simulink model "BerylMambo"  (R2019b)
settings: Solver=FixedStepAuto  StartTime=0.0  StopTime=100  FixedStep=1/200  RelTol=1e-3
InitFcn:
  | load('BusDefinitions.mat')
undefined symbols (not defined in the file or in its folder): codertarget, DiscIntNeverNeededParam, Discrete, sigbuilder_block, Time
libraries: dspstat3 x7, simulink x5, parrotlib x2, ctrlSharedLib x1
settings Model: SimulationMode=external  ExtModeTrigDuration=80  Creator=kelvinxie  LastModifiedBy=kelvinxie
settings OptimizationCC: PassReuseOutputArgsThreshold=0  MaxStackSize=64  SimCompilerOptimization=on
settings DebuggingCC: ParameterTunabilityLossMsg=error  ArithmeticOperatorsInVariantConditions=warning
settings HardwareCC: ProdBitPerPointer=32  ProdBitPerSizeT=32  ProdBitPerPtrDiffT=32  ProdLargestAtomicInteger=Long  ProdWordSize=32  ProdHWDeviceType=ARM Compatible->ARM 9
settings SFSimCC: SimUseLocalCustomCode=off  MATLABDynamicMemAlloc=off
settings RTWCC: SystemTargetFile=ert.tlc  HardwareBoard=PARROT Mambo  TLCOptions="-aInlineSetEventsForThisBaseRateFcn=TLC_FALSE -aSuppressMultiTaskScheduler=TLC_FALSE   -aRateBasedStepFcn=1"  TemplateMakefile=ert_default_tmf  GenerateReport=on  RTWVerbose=off  RTWUseLocalCustomCode=off  Toolchain=Sourcery G++ Lite GNU Toolchain for Drones  BuildConfiguration=Faster Runs
settings CodeAppCC: ForceParamTrailComments=on  OperatorAnnotations=on  StateflowObjectComments=on
settings ERTTargetCC: ERTCustomFileBanners=off  MatFileLogging=on  SupportContinuousTime=on  SupportNonInlinedSFcns=on  RemoveResetFunc=off  ModelStepFunctionPrototypeControlCompliant=off

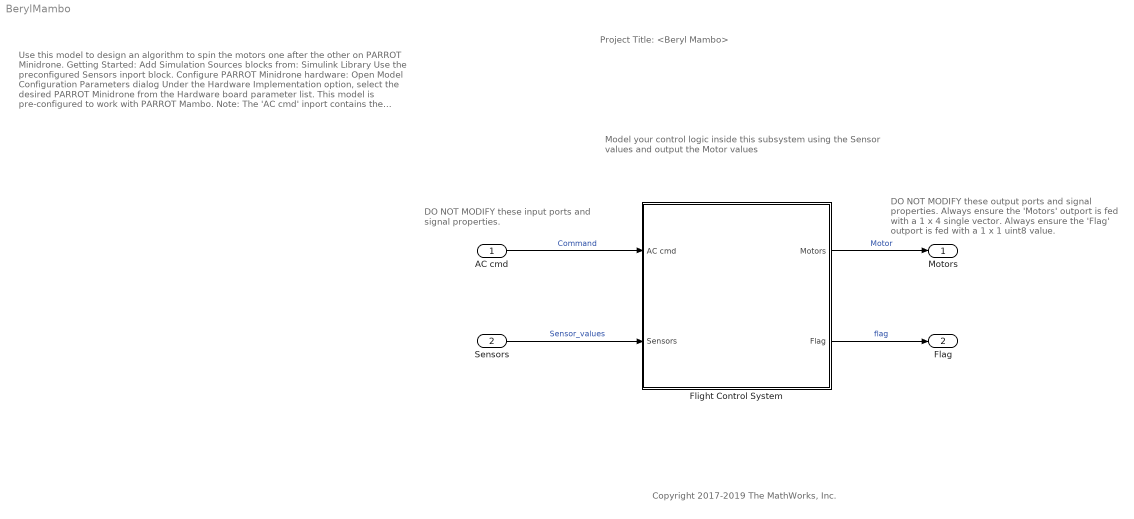
== system BerylMambo ==
  note: Model your control logic inside this subsystem
      | using the Sensor values and output the
      | Motor values
  note: DO NOT MODIFY these output ports
      | and signal properties.
      |
      |
      |
      | Always ensure the 'Motors' outport
      | is fed with a 1 x 4 single vector.
      |
      |
      |
      |
      |
      | Always ensure the 'Flag' outport is
      | fed with a 1 x 1 uint8 value.
  note: DO NOT MODIFY these input
      | ports and signal properties.
  note: Copyright 2017-2019 The MathWorks, Inc.
  note: Use this model to design an algorithm to spin the motors one
      | after the other on PARROT Minidrone.
      |
      | Getting Started:
      |
      | Add Simulation Sources blocks from:
      | Simulink Library
      | Use the preconfigured Sensors inport block.
      |
      | Configure PARROT Minidrone hardware:
      |
      | Open Model Configuration Parameters dialog
      |
      | Under the Hardware Implementation option, select the desired
      | PARROT Minidrone from the Hardware board parameter list.
      |
      | This model is pre-configured to work with PARROT Mambo.
      |
      | Note:
      |
      | The 'AC cmd' inport contains the position and orientation
      | reference signals information.
      | The 'Sensors' inport contains data from accelerometer,
      | gyroscope, ultrasonic, pressure and optical flow data.
      | The 'Flag' outport can be used to model an error condition
      | which stops the drone.
      | The 'Motors' outport is fed with the speed values of the 4 motors.
      | Learn more:
      |
      | Simulink Subsystem
      | Simulink Buses
  note: Project Title: <Beryl Mambo>
  AC cmd : Inport  OutDataTypeStr=Bus: CommandBus  BusOutputAsStruct=on
  Sensors : Inport  Port=2  OutDataTypeStr=Bus: SensorsBus  BusOutputAsStruct=on
  Flight Control System : Subsystem  InitFcn=codertarget.parrot.internal.fcsSubsystemCallback(gcb);
  Motors : Outport  OutDataTypeStr=single  PortDimensions=[1 4]  VectorParamsAs1DForOutWhenUnconnected=off
  Flag : Outport  Port=2  OutDataTypeStr=uint8  PortDimensions=1  VectorParamsAs1DForOutWhenUnconnected=off
  wires:
  Flight Control System/1(Motors) -> Motors/1  "Motor"
  AC cmd/1 -> Flight Control System/1(AC cmd)  "Command"
  Sensors/1 -> Flight Control System/2(Sensors)  "Sensor_values"
  Flight Control System/2(Flag) -> Flag/1  "flag"

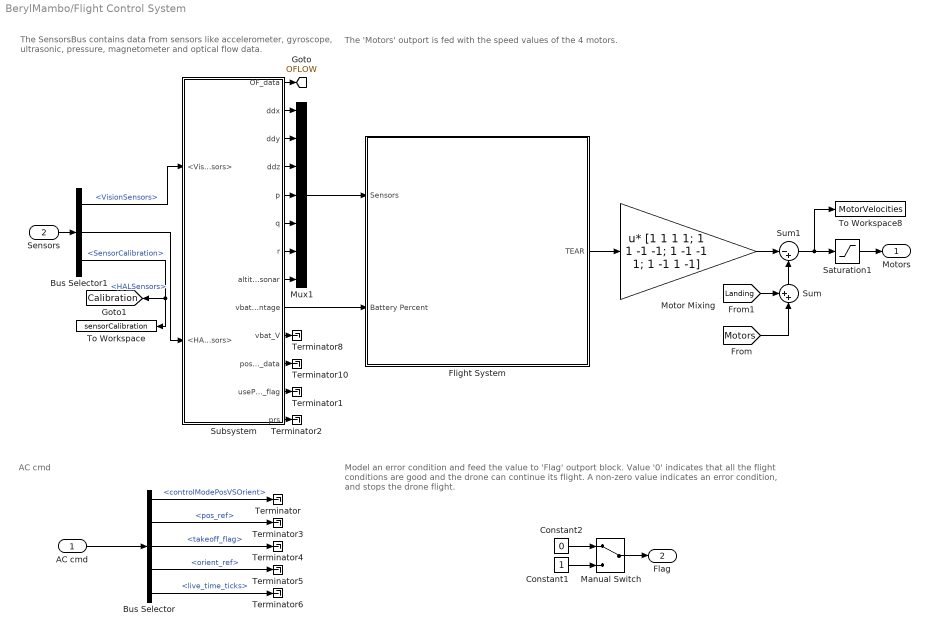
== system BerylMambo/Flight Control System ==
  note: AC cmd
  note: The 'Motors' outport is fed with the speed values of the 4 motors.
  note: Model an error condition and feed the value to 'Flag' outport block. Value '0' indicates that all the flight conditions are
      | good and the drone can continue its flight. A non-zero value indicates an error condition, and stops the drone flight.
  note: The SensorsBus contains data from sensors like
      | accelerometer, gyroscope, ultrasonic, pressure,
      | magnetometer and optical flow data.
  AC cmd : Inport
  Sensors : Inport  Port=2
  Bus Selector : BusSelector  OutputSignals=controlModePosVSOrient,pos_ref,takeoff_flag,orient_ref,live_time_ticks
  Bus Selector1 : BusSelector  OutputSignals=VisionSensors,HALSensors,SensorCalibration
  Constant1 : Constant  OutDataTypeStr=uint8
  Constant2 : Constant  Value=0  OutDataTypeStr=uint8
  Flight System : Subsystem
  Manual Switch : ManualSwitch
  "Motor Mixing            " : Gain  Gain=[1 1 1 1; 1 1 -1 -1; 1 -1 -1 1; 1 -1 1 -1]  Multiplication=Matrix(u*K)
  Mux1 : Mux  Inputs=7
  Saturation1 : Saturate  UpperLimit=500  LowerLimit=0  OutDataTypeStr=single
  Subsystem : Subsystem
  Sum : Sum  Inputs=++|
  Sum1 : Sum  Inputs=|-+  OutDataTypeStr=single
  Terminator{,1..6,8,10} (9 alike) : Terminator
  To Workspace : ToWorkspace  VariableName=sensorCalibration  SaveFormat=Structure With Time  SampleTime=-1
  To Workspace8 : ToWorkspace  VariableName=MotorVelocities  SaveFormat=Structure With Time  SampleTime=-1
  Motors : Outport  VectorParamsAs1DForOutWhenUnconnected=off
  Flag : Outport  Port=2  VectorParamsAs1DForOutWhenUnconnected=off
  tag scope: Calibration=global, OFLOW=global
  wires:
  AC cmd/1 -> Bus Selector/1
  Sensors/1 -> Bus Selector1/1
  Bus Selector/1 -> Terminator/1  "<controlModePosVSOrient>"
  Bus Selector/2 -> Terminator3/1  "<pos_ref>"
  Bus Selector/3 -> Terminator4/1  "<takeoff_flag>"
  Bus Selector/4 -> Terminator5/1  "<orient_ref>"
  Bus Selector/5 -> Terminator6/1  "<live_time_ticks>"
  Manual Switch/1 -> Flag/1
  Constant2/1 -> Manual Switch/1
  Constant1/1 -> Manual Switch/2
  Saturation1/1 -> Motors/1
  Bus Selector1/1 -> Subsystem/1(<VisionSensors>)  "<VisionSensors>"
  Bus Selector1/2 -> Subsystem/2(<HALSensors>)  "<HALSensors>"
  Bus Selector1/3 -> To Workspace/1, [Calibration]  "<SensorCalibration>"
  Subsystem/11(posVIS_data) -> Terminator10/1
  Subsystem/12(usePosVIS_flag) -> Terminator1/1
  Subsystem/13(prs) -> Terminator2/1
  Subsystem/9(vbat_percentage) -> Flight System/2(Battery Percent)
  Subsystem/10(vbat_V) -> Terminator8/1
  Flight System/1("TEAR ") -> "Motor Mixing            "/1
  Mux1/1 -> Flight System/1(Sensors)
  Subsystem/7(r) -> Mux1/6
  Subsystem/6(q) -> Mux1/5
  Subsystem/8(altitude_sonar) -> Mux1/7
  Subsystem/5(p) -> Mux1/4
  Subsystem/4(ddz) -> Mux1/3
  Subsystem/3(ddy) -> Mux1/2
  Subsystem/2(ddx) -> Mux1/1
  Subsystem/1(OF_data) -> [OFLOW]
  "Motor Mixing            "/1 -> Sum1/1
  Sum/1 -> Sum1/2
  [Landing] -> Sum/1
  [Motors] -> Sum/2
  Sum1/1 -> Saturation1/1, To Workspace8/1

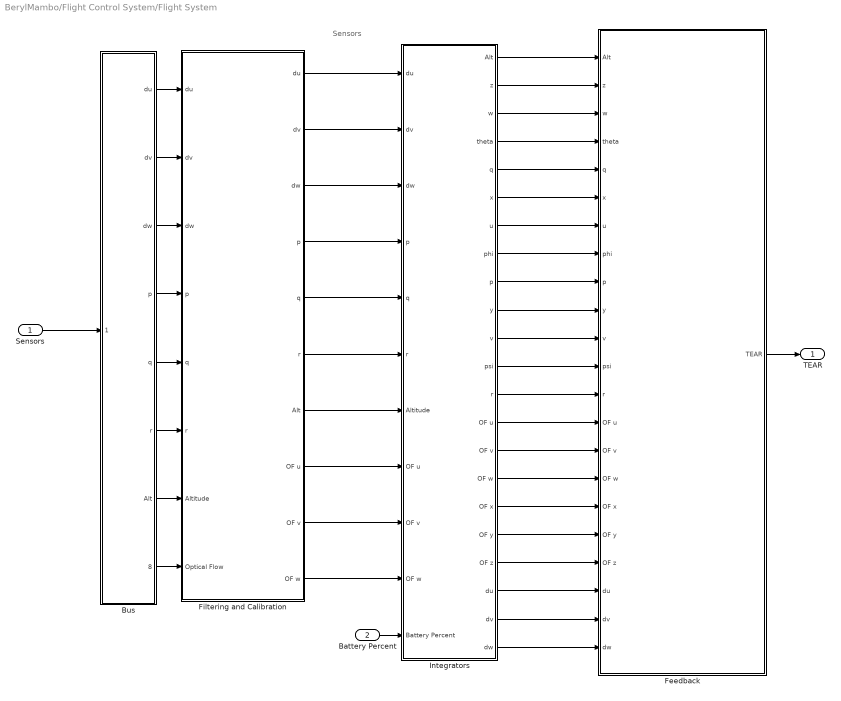
== system BerylMambo/Flight Control System/Flight System ==
  note: Sensors
  Sensors : Inport
  Battery Percent : Inport  Port=2
  Bus : Subsystem
  Feedback : Subsystem
  Filtering and Calibration : Subsystem
  Integrators : Subsystem
  "TEAR " : Outport
  wires:
  Battery Percent/1 -> Integrators/11(Battery Percent)
  Filtering and Calibration/1("du ") -> Integrators/1(du)
  Filtering and Calibration/2("dv ") -> Integrators/2(dv)
  Filtering and Calibration/3("dw ") -> Integrators/3(dw)
  Filtering and Calibration/4("p ") -> Integrators/4(p)
  Filtering and Calibration/5("q ") -> Integrators/5(q)
  Filtering and Calibration/6("r ") -> Integrators/6(r)
  Filtering and Calibration/7(Alt) -> Integrators/7(Altitude)
  Bus/7(Alt) -> Filtering and Calibration/7(Altitude)
  Bus/6(r) -> Filtering and Calibration/6(r)
  Bus/5(q) -> Filtering and Calibration/5(q)
  Bus/4(p) -> Filtering and Calibration/4(p)
  Bus/3(dw) -> Filtering and Calibration/3(dw)
  Bus/2(dv) -> Filtering and Calibration/2(dv)
  Bus/1(du) -> Filtering and Calibration/1(du)
  Sensors/1 -> Bus/1(Sensors)
  Bus/8(Optical Flow) -> Filtering and Calibration/8(Optical Flow)
  Filtering and Calibration/8("OF u ") -> Integrators/8("OF u ")
  Filtering and Calibration/9("OF v ") -> Integrators/9("OF v ")
  Filtering and Calibration/10("OF w ") -> Integrators/10("OF w ")
  Feedback/1("TEAR ") -> "TEAR "/1
  Integrators/1("Alt ") -> Feedback/1(Alt)
  Integrators/2("z ") -> Feedback/2("z ")
  Integrators/3("w ") -> Feedback/3("w ")
  Integrators/4("theta ") -> Feedback/4("theta ")
  Integrators/5("q ") -> Feedback/5(q)
  Integrators/6("x ") -> Feedback/6("x ")
  Integrators/7("u ") -> Feedback/7("u ")
  Integrators/8("phi ") -> Feedback/8("phi ")
  Integrators/9("p ") -> Feedback/9(p)
  Integrators/10("y ") -> Feedback/10("y ")
  Integrators/11("v ") -> Feedback/11("v ")
  Integrators/12("psi ") -> Feedback/12(psi)
  Integrators/13("r ") -> Feedback/13(r)
  Integrators/14(OF u) -> Feedback/14(OF u)
  Integrators/15("OF v ") -> Feedback/15(OF v)
  Integrators/16(OF w) -> Feedback/16(OF w)
  Integrators/17("OF x ") -> Feedback/17(OF x)
  Integrators/18("OF y ") -> Feedback/18(OF y)
  Integrators/19("OF z ") -> Feedback/19(OF z)
  Integrators/20("du ") -> Feedback/20(du)
  Integrators/21("dv ") -> Feedback/21(dv)
  Integrators/22("dw ") -> Feedback/22(dw)

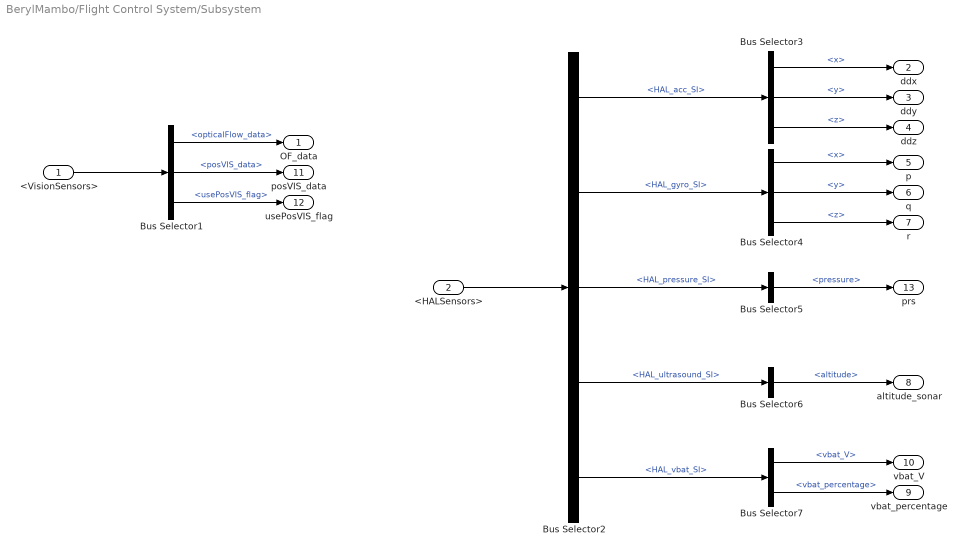
== system BerylMambo/Flight Control System/Subsystem ==
  <VisionSensors> : Inport
  <HALSensors> : Inport  Port=2
  Bus Selector1 : BusSelector  OutputSignals=opticalFlow_data,posVIS_data,usePosVIS_flag
  Bus Selector2 : BusSelector  OutputSignals=HAL_acc_SI,HAL_gyro_SI,HAL_pressure_SI,HAL_ultrasound_SI,HAL_vbat_SI
  Bus Selector3 : BusSelector  OutputSignals=x,y,z
  Bus Selector4 : BusSelector  OutputSignals=x,y,z
  Bus Selector5 : BusSelector  OutputSignals=pressure
  Bus Selector6 : BusSelector  OutputSignals=altitude
  Bus Selector7 : BusSelector  OutputSignals=vbat_V,vbat_percentage
  OF_data : Outport  VectorParamsAs1DForOutWhenUnconnected=off
  ddx : Outport  Port=2  VectorParamsAs1DForOutWhenUnconnected=off
  ddy : Outport  Port=3  VectorParamsAs1DForOutWhenUnconnected=off
  ddz : Outport  Port=4  VectorParamsAs1DForOutWhenUnconnected=off
  p : Outport  Port=5  VectorParamsAs1DForOutWhenUnconnected=off
  q : Outport  Port=6  VectorParamsAs1DForOutWhenUnconnected=off
  r : Outport  Port=7  VectorParamsAs1DForOutWhenUnconnected=off
  altitude_sonar : Outport  Port=8  VectorParamsAs1DForOutWhenUnconnected=off
  vbat_percentage : Outport  Port=9  VectorParamsAs1DForOutWhenUnconnected=off
  vbat_V : Outport  Port=10  VectorParamsAs1DForOutWhenUnconnected=off
  posVIS_data : Outport  Port=11  VectorParamsAs1DForOutWhenUnconnected=off
  usePosVIS_flag : Outport  Port=12  VectorParamsAs1DForOutWhenUnconnected=off
  prs : Outport  Port=13  VectorParamsAs1DForOutWhenUnconnected=off
  wires:
  <VisionSensors>/1 -> Bus Selector1/1
  <HALSensors>/1 -> Bus Selector2/1
  Bus Selector1/1 -> OF_data/1  "<opticalFlow_data>"
  Bus Selector1/2 -> posVIS_data/1  "<posVIS_data>"
  Bus Selector1/3 -> usePosVIS_flag/1  "<usePosVIS_flag>"
  Bus Selector2/1 -> Bus Selector3/1  "<HAL_acc_SI>"
  Bus Selector2/2 -> Bus Selector4/1  "<HAL_gyro_SI>"
  Bus Selector2/3 -> Bus Selector5/1  "<HAL_pressure_SI>"
  Bus Selector2/4 -> Bus Selector6/1  "<HAL_ultrasound_SI>"
  Bus Selector2/5 -> Bus Selector7/1  "<HAL_vbat_SI>"
  Bus Selector3/1 -> ddx/1  "<x>"
  Bus Selector3/2 -> ddy/1  "<y>"
  Bus Selector3/3 -> ddz/1  "<z>"
  Bus Selector4/2 -> q/1  "<y>"
  Bus Selector4/1 -> p/1  "<x>"
  Bus Selector4/3 -> r/1  "<z>"
  Bus Selector5/1 -> prs/1  "<pressure>"
  Bus Selector6/1 -> altitude_sonar/1  "<altitude>"
  Bus Selector7/1 -> vbat_V/1  "<vbat_V>"
  Bus Selector7/2 -> vbat_percentage/1  "<vbat_percentage>"

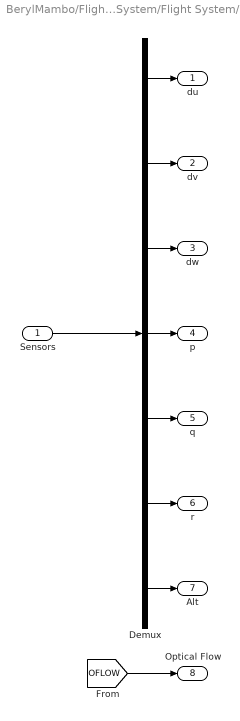
== system BerylMambo/Flight Control System/Flight System/Bus ==
  Sensors : Inport
  Demux : Demux  Outputs=7
  du : Outport
  dv : Outport  Port=2
  dw : Outport  Port=3
  p : Outport  Port=4
  q : Outport  Port=5
  r : Outport  Port=6
  Alt : Outport  Port=7
  Optical Flow : Outport  Port=8
  wires:
  Sensors/1 -> Demux/1
  Demux/7 -> Alt/1
  Demux/6 -> r/1
  Demux/5 -> q/1
  Demux/4 -> p/1
  Demux/3 -> dw/1
  Demux/2 -> dv/1
  Demux/1 -> du/1
  [OFLOW] -> Optical Flow/1

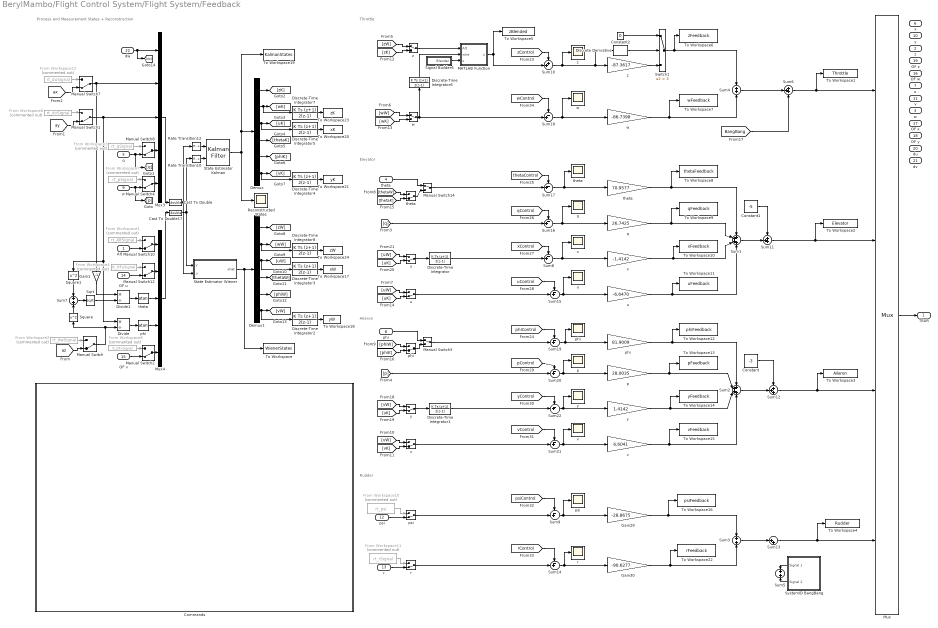
== system BerylMambo/Flight Control System/Flight System/Feedback ==
  note: Process and Measurement States + Reconstruction
  note: Rudder
  note: Aileron
  note: Elevator
  note: Throttle
  Alt : Inport
  "z " : Inport  Port=2
  "w " : Inport  Port=3
  "theta " : Inport  Port=4
  q : Inport  Port=5
  "x " : Inport  Port=6
  "u " : Inport  Port=7
  "phi " : Inport  Port=8
  p : Inport  Port=9
  "y " : Inport  Port=10
  "v " : Inport  Port=11
  psi : Inport  Port=12
  r : Inport  Port=13
  OF u : Inport  Port=14
  OF v : Inport  Port=15
  OF w : Inport  Port=16
  OF x : Inport  Port=17
  OF y : Inport  Port=18
  OF z : Inport  Port=19
  du : Inport  Port=20
  dv : Inport  Port=21
  dw : Inport  Port=22
  Cast To Double : DataTypeConversion  OutDataTypeStr=double
  Cast To Double17 : DataTypeConversion  OutDataTypeStr=double
  "Commands " : Subsystem
  Constant : Constant  Value=-3
  Constant1 : Constant  Value=-5
  Constant2 : Constant  Value=0
  Demux : Demux  Outputs=6
  Demux1 : Demux  Outputs=6
  Discrete Derivative : simulink/Discrete/Discrete Derivative  gainval=1.0  ICPrevScaledInput=0.0  OutMin=[]  OutMax=[]  OutDataType=fixdt(1, 16)  OutScaling=2^-10  DoSatur=off
  Discrete-Time Integrator{,1..8} (9 alike) : DiscreteIntegrator  IntegratorMethod=Integration: Trapezoidal  SampleTime=1/200  ICPrevOutput=DiscIntNeverNeededParam  ICPrevScaledInput=DiscIntNeverNeededParam
  Divide : Product  Inputs=*/
  Divide1 : Product  Inputs=*/
  From Workspace1 : FromWorkspace  Commented=on  VariableName=rt_AltSignal  SampleTime=0
  From Workspace10 : FromWorkspace  Commented=on  VariableName=rt_psi  SampleTime=0
  From Workspace11 : FromWorkspace  Commented=on  VariableName=rt_rSignal  SampleTime=0
  From Workspace12 : FromWorkspace  Commented=on  VariableName=rt_duSignal  SampleTime=0
  From Workspace2 : FromWorkspace  Commented=on  VariableName=rt_dwSignal  SampleTime=0
  From Workspace3 : FromWorkspace  Commented=on  VariableName=rt_qSignal  SampleTime=0
  From Workspace4 : FromWorkspace  Commented=on  VariableName=rt_OFuSignal  SampleTime=0
  From Workspace6 : FromWorkspace  Commented=on  VariableName=rt_dvSignal  SampleTime=0
  From Workspace7 : FromWorkspace  Commented=on  VariableName=rt_pSignal  SampleTime=0
  From Workspace8 : FromWorkspace  Commented=on  VariableName=rt_OFvSignal  SampleTime=0
  Gain1 : Gain  Gain=-1
  Gain29 : Gain  Gain=-28.8675
  Gain30 : Gain  Gain=-90.6277
  MATLAB Function : MATLAB Function  TreatAsAtomicUnit=on
  Manual Switch{,1..2,4,7..8,10,12} (8 alike) : ManualSwitch  CurrentSetting=0
  Manual Switch14 : ManualSwitch
  Manual Switch3 : ManualSwitch
  Mux : Mux
  Mux3 : Mux  Inputs=5
  Mux4 : Mux  Inputs=5
  Rate Transition10 : RateTransition  OutPortSampleTimeOpt=Inherit  OutPortSampleTime=1/200
  Rate Transition12 : RateTransition  OutPortSampleTimeOpt=Inherit  OutPortSampleTime=1/200
  Reconstructed States : Scope
  Signal Builder6 : Subsystem  Tag=STV Subsys  LoadFcn=sigbuilder_block('load');  StartFcn=sigbuilder_block('start');  StopFcn=sigbuilder_block('stop');  ClipboardFcn=sigbuilder_block('clipboard');  mask(Sigbuilder block){tuvar=[0:10]}
      mask help: Simulink:masks:SigbuilderBlock_MD
      mask init:
      | if ~strcmp(get_param(bdroot(gcbh),'SimulationStatus'),'stopped') tuvar = sigbuilder_block('maskInit'); end
      settings: CopyFcn=sigbuilder_block('copy');  DeleteFcn=sigbuilder_block('delete');  ModelCloseFcn=sigbuilder_block('modelClose');  PreSaveFcn=sigbuilder_block('preSave');  PauseFcn=sigbuilder_block('pause');  ContinueFcn=sigbuilder_block('continue');  NameChangeFcn=sigbuilder_block('namechange');  OpenFcn=sigbuilder_block('open',[437.6 199.2 550.4 400 ]);  CloseFcn=sigbuilder_block('close');
      mask Display: plot(0, 0, 100, 100,[2, 2, 32, 32, 2], [68, 8, 8, 68, 68],[32, 2], [38, 38], [32, 19, 2],[53, 60, 44], [32, 17, 17, 2],[16, 16, 31, 31]);txt = getActiveGroup(gcbh);text(2, 100, txt,'verticalAlignment', 'top');
  Sqrt : Sqrt  SaturateOnIntegerOverflow=on
  Square : Math  Operator=square  SignedPower=off  SaturateOnIntegerOverflow=on
  Square1 : Math  Operator=square  SignedPower=off  SaturateOnIntegerOverflow=on
  State Estimator Kalman : ctrlSharedLib/Kalman Filter  TimeDomain=Discrete-Time  UseCurrentEstimator=on  ModelSource=Individual A, B, C, D matrices  ModelSourceVariable=ss(0.95,1,1,0,1)  A=|  B=|  C=|  D=0  NumberOfStates=1  NumberOfInputs=1  NumberOfOutputs=1  InitialEstimateSource=Dialog  X0=0  P0=10  UseK=off  UseGH=off  NumberOfProcessNoiseInputs=1  G=1  TimeInvariantG=on  H=0  TimeInvariantH=on  Q=[0,0,0,0,0,0;0,0.0103299030000000,-0.00175759940000000,0.000594682880000000,0.000181117150000000,-7.39573080000000e-05;0,-0.00175759940000000,0.0118374790000000,-0.00221546480000000,-5.20388240000000e-05,0.000234450610000000;0,0.000594682880000000,-0.00221546480000000,0.0200744810000000,-0.000197027910000000,0.000332269530000000;0,0.000181117150000000,-5.20388240000000e-05,-0.000197027910000000,0.00104430880000000,-1.70153140000000e-05;0,-7.39573080000000e-05,0.000234450610000000,0.000332269530000000,-1.70153140000000e-05,0.000900396260000000]  TimeInvariantQ=on  R=[0.00202988690000000,3.86984470000000e-05,1.00000000000000e-08,0.00305777280000000,1.00000000000000e-08;3.86984470000000e-05,0.000833637900000000,1.00000000000000e-08,0.00208964520000000,1.00000000000000e-08;1.00000000000000e-08,1.00000000000000e-08,48.8126395000000,1.00000000000000e-08,0.00164671100000000;0.00305777280000000,0.00208964520000000,1.00000000000000e-08,27.7868240000000,0.000704304490000000;1.00000000000000e-08,1.00000000000000e-08,0.00164671100000000,0.000704304490000000,0.000587063430000000]  TimeInvariantR=on  N=0  TimeInvariantN=on  AddInputPort=on  AddEnablePort=off  OutputEstimatedY=off  OutputP=off  Ts=1/200
      A=|
      | [1.0000    0.0050         0         0         0         0;
      |          0    1.0000         0         0         0         0;
      |          0         0    1.0000         0         0         0;
      |          0         0         0    1.0000         0         0;
      |          0         0         0         0    1.0000         0;
      |          0         0         0         0         0    1.0000]
      B=|
      | [0.0000         0         0         0         0;
      |     0.0050         0         0         0         0;
      |          0    0.0050         0         0         0;
      |          0         0         0    0.0050         0;
      |          0         0         0         0    0.0050;
      |          0         0    0.0050         0         0]
      C=|
      | [-1 0 0 0 0 0;
      |       0 0 1 0 0 0;
      |       0 0 0 1 0 0;
      |       0 0 0 0 1 0;
      |       0 0 0 0 0 1]
      settings: SourceProductBaseCode=CT
  "State Estimator Wiener " : Subsystem
  Sum1 : Sum  Inputs=++++  OutDataTypeStr=single
  Sum10 : Sum  Inputs=++|
  Sum11 : Sum  Inputs=+++  AccumDataTypeStr=single  OutDataTypeStr=single
  Sum12 : Sum  Inputs=+++  OutDataTypeStr=single
  Sum13 : Sum  Inputs=|++  OutDataTypeStr=single
  Sum{8..9,14..15,17..19,21..22} (9 alike) : Sum  Inputs=-+|
  Sum16 : Sum  Inputs=-+|  OutDataTypeStr=double
  Sum2 : Sum  Inputs=++++  OutDataTypeStr=single
  Sum20 : Sum  Inputs=-+|  OutDataTypeStr=double
  Sum3 : Sum
  Sum4 : Sum  Inputs=+|+  OutDataTypeStr=single
  Sum5 : Sum  OutDataTypeStr=single
  Sum6 : Sum  Inputs=+++  OutDataTypeStr=single
  Sum7 : Sum
  Switch1 : Switch  Criteria=u2 > Threshold  Threshold=3
  SystemID BangBang : Subsystem  Tag=STV Subsys  LoadFcn=sigbuilder_block('load');  StartFcn=sigbuilder_block('start');  StopFcn=sigbuilder_block('stop');  ClipboardFcn=sigbuilder_block('clipboard');  mask(Sigbuilder block){tuvar=[0:10]}
      mask help: Simulink:masks:SigbuilderBlock_MD
      mask init:
      | if ~strcmp(get_param(bdroot(gcbh),'SimulationStatus'),'stopped') tuvar = sigbuilder_block('maskInit'); end
      settings: CopyFcn=sigbuilder_block('copy');  DeleteFcn=sigbuilder_block('delete');  ModelCloseFcn=sigbuilder_block('modelClose');  PreSaveFcn=sigbuilder_block('preSave');  PauseFcn=sigbuilder_block('pause');  ContinueFcn=sigbuilder_block('continue');  NameChangeFcn=sigbuilder_block('namechange');  OpenFcn=sigbuilder_block('open',[153 118 1287 686 ]);  CloseFcn=sigbuilder_block('close');
      mask Display: plot(0, 0, 100, 100,[2, 2, 32, 32, 2], [68, 8, 8, 68, 68],[32, 2], [38, 38], [32, 19, 2],[53, 60, 44], [32, 17, 17, 2],[16, 16, 31, 31]);txt = getActiveGroup(gcbh);text(2, 100, txt,'verticalAlignment', 'top');
  To Workspace : ToWorkspace  VariableName=WienerStates  SaveFormat=Structure With Time  SampleTime=-1
  To Workspace1 : ToWorkspace  VariableName=Throttle  SaveFormat=Structure With Time  SampleTime=-1
  To Workspace10 : ToWorkspace  VariableName=xFeedback  SaveFormat=Structure With Time  SampleTime=-1
  To Workspace11 : ToWorkspace  VariableName=uFeedback  SaveFormat=Structure With Time  SampleTime=-1
  To Workspace12 : ToWorkspace  VariableName=phiFeedback  SaveFormat=Structure With Time  SampleTime=-1
  To Workspace13 : ToWorkspace  VariableName=pFeedback  SaveFormat=Structure With Time  SampleTime=-1
  To Workspace14 : ToWorkspace  VariableName=yFeedback  SaveFormat=Structure With Time  SampleTime=-1
  To Workspace15 : ToWorkspace  VariableName=vFeedback  SaveFormat=Structure With Time  SampleTime=-1
  To Workspace16 : ToWorkspace  VariableName=psiFeedback  SaveFormat=Structure With Time  SampleTime=-1
  To Workspace17 : ToWorkspace  VariableName=xW  SaveFormat=Structure With Time  SampleTime=-1
  To Workspace18 : ToWorkspace  VariableName=yW  SaveFormat=Structure With Time  SampleTime=-1
  To Workspace19 : ToWorkspace  VariableName=KalmanStates  SaveFormat=Structure With Time  SampleTime=-1
  To Workspace2 : ToWorkspace  VariableName=Elevator  SaveFormat=Structure With Time  SampleTime=-1
  To Workspace20 : ToWorkspace  VariableName=xK  SaveFormat=Structure With Time  SampleTime=-1
  To Workspace21 : ToWorkspace  VariableName=yK  SaveFormat=Structure With Time  SampleTime=-1
  To Workspace22 : ToWorkspace  VariableName=rFeedback  SaveFormat=Structure With Time  SampleTime=-1
  To Workspace23 : ToWorkspace  VariableName=zK  SaveFormat=Structure With Time  SampleTime=-1
  To Workspace24 : ToWorkspace  VariableName=zW  SaveFormat=Structure With Time  SampleTime=-1
  To Workspace3 : ToWorkspace  VariableName=Aileron  SaveFormat=Structure With Time  SampleTime=-1
  To Workspace4 : ToWorkspace  VariableName=Rudder  SaveFormat=Structure With Time  SampleTime=-1
  To Workspace5 : ToWorkspace  VariableName=zBlended  SaveFormat=Structure With Time  SampleTime=-1
  To Workspace6 : ToWorkspace  VariableName=zFeedback  SaveFormat=Structure With Time  SampleTime=-1
  To Workspace7 : ToWorkspace  VariableName=wFeedback  SaveFormat=Structure With Time  SampleTime=-1
  To Workspace8 : ToWorkspace  VariableName=thetaFeedback  SaveFormat=Structure With Time  SampleTime=-1
  To Workspace9 : ToWorkspace  VariableName=qFeedback  SaveFormat=Structure With Time  SampleTime=-1
  "p " : Gain  Gain=28.0035
  "p " : Scope
  phi : Gain  Gain=81.9009
  "phi " : Scope
  "phi " : Trigonometry  Operator=atan
  "phi " : ManualSwitch  CurrentSetting=0
  "psi " : Scope
  "psi " : ManualSwitch  CurrentSetting=0
  "q " : Gain  Gain=26.7425
  "q " : Scope
  "r " : Scope
  "r " : ManualSwitch  CurrentSetting=0
  theta : Gain  Gain=70.9577
  "theta " : Scope
  "theta " : Trigonometry  Operator=atan
  "theta " : ManualSwitch  CurrentSetting=0
  u : Gain  Gain=-6.6470
  "u " : Scope
  "u " : ManualSwitch  CurrentSetting=0
  v : Gain  Gain=6.6041
  "v " : Scope
  "v " : ManualSwitch  CurrentSetting=0
  w : Gain  Gain=-86.7398
  "w " : Scope
  "w " : ManualSwitch
  x : Gain  Gain=-1.4142
  "x " : Scope
  "x " : ManualSwitch  CurrentSetting=0
  y : Gain  Gain=1.4142
  "y " : Scope
  "y " : ManualSwitch  CurrentSetting=0
  z : Gain  Gain=-87.3617
  "z " : Scope
  "z " : ManualSwitch
  "TEAR " : Outport
  wires:
  Gain1/1 -> Divide1/1
  Alt/1 -> Manual Switch10/2
  "r "/1 -> Sum14/2
  v/1 -> To Workspace15/1, Sum2/4
  Sum7/1 -> Sqrt/1
  Sum3/1 -> Sum13/1
  From Workspace6/1 -> Manual Switch1/1
  Divide1/1 -> "theta "/1
  q/1 -> Manual Switch8/2, [q]
  From Workspace7/1 -> Manual Switch4/1
  Gain29/1 -> To Workspace16/1, Sum3/1
  phi/1 -> To Workspace12/1, Sum2/1
  "psi "/1 -> Sum9/2
  From Workspace10/1 -> "psi "/1
  Sum4/1 -> Sum6/2
  Divide/1 -> "phi "/1
  Square/1 -> Sum7/2
  From Workspace3/1 -> Manual Switch8/1
  Switch1/1 -> To Workspace6/1, Sum4/1
  "p "/1 -> Sum2/2, To Workspace13/1
  Sqrt/1 -> Divide1/2
  w/1 -> Sum4/2, To Workspace7/1
  Sum10/1 -> z/1, Discrete Derivative/1, "z "/1
  From Workspace8/1 -> Manual Switch2/1
  Sum1/1 -> Sum11/2
  Square1/1 -> Sum7/1
  Manual Switch12/1 -> Mux4/2
  From Workspace2/1 -> Manual Switch/1
  p/1 -> [p], Manual Switch4/2
  y/1 -> To Workspace14/1, Sum2/3
  Mux/1 -> "TEAR "/1
  Gain30/1 -> To Workspace22/1, Sum3/2
  r/1 -> "r "/2
  From Workspace1/1 -> Manual Switch10/1
  psi/1 -> "psi "/2
  From Workspace4/1 -> Manual Switch12/1
  From Workspace11/1 -> "r "/1
  From Workspace12/1 -> Manual Switch7/1
  Sum12/1 -> Mux/3, To Workspace3/1
  Sum11/1 -> Mux/2, To Workspace2/1
  Sum13/1 -> Mux/4, To Workspace4/1
  "phi "/1 -> Manual Switch3/1
  "theta "/1 -> Mux4/3
  "phi "/1 -> Mux4/4
  Manual Switch10/1 -> Mux4/1
  Manual Switch2/1 -> Mux4/5
  Mux3/1 -> Cast To Double/1
  Mux4/1 -> Cast To Double17/1
  Manual Switch4/1 -> Mux3/5
  Manual Switch8/1 -> Mux3/4
  Manual Switch1/1 -> Mux3/3, Square1/1, Divide/1
  Manual Switch7/1 -> Mux3/2, Gain1/1
  Manual Switch/1 -> Square/1, Divide/2
  Cast To Double/1 -> "State Estimator Wiener "/2(u), Rate Transition12/1
  Cast To Double17/1 -> "State Estimator Wiener "/1(y), Rate Transition10/1
  State Estimator Kalman/1 -> Reconstructed States/1, To Workspace19/1, Demux/1
  Discrete-Time Integrator1/1 -> Sum22/2
  [p] -> Sum20/2
  "State Estimator Wiener "/1(xhat) -> Demux1/1, To Workspace/1
  Rate Transition12/1 -> State Estimator Kalman/1
  Rate Transition10/1 -> State Estimator Kalman/2
  OF u/1 -> Manual Switch12/2
  OF v/1 -> Manual Switch2/2
  [az] -> Manual Switch/2
  dw/1 -> [dw], Mux3/1
  [ax] -> Manual Switch7/2
  [ay] -> Manual Switch1/2
  Discrete-Time Integrator3/1 -> To Workspace17/1
  Discrete-Time Integrator2/1 -> To Workspace18/1
  Demux/1 -> [zK]
  Demux/2 -> Discrete-Time Integrator7/1, [wK]
  Demux/6 -> Discrete-Time Integrator4/1, [vK]
  Demux/5 -> [phiK]
  Demux/4 -> [thetaK]
  Demux1/2 -> Discrete-Time Integrator8/1, [wW]
  Demux1/4 -> [thetaW]
  Demux1/1 -> [zW]
  Demux1/5 -> [phiW]
  Demux1/3 -> Discrete-Time Integrator3/1, [uW]
  Demux1/6 -> Discrete-Time Integrator2/1, [vW]
  [zW] -> "z "/1
  [zK] -> "z "/2
  "w "/1 -> Sum18/2, Discrete-Time Integrator6/1
  [wK] -> "w "/2
  [wW] -> "w "/1
  [phiK] -> "phi "/2
  [phiW] -> "phi "/1
  [vK] -> "v "/2
  [vW] -> "v "/1
  "v "/1 -> Sum21/2
  Discrete-Time Integrator4/1 -> To Workspace21/1
  Discrete-Time Integrator5/1 -> To Workspace20/1
  Demux/3 -> Discrete-Time Integrator5/1, [uK]
  Discrete-Time Integrator7/1 -> To Workspace23/1
  Discrete-Time Integrator8/1 -> To Workspace24/1
  Sum6/1 -> Mux/1, To Workspace1/1
  MATLAB Function/1(z) -> Sum10/2, To Workspace5/1
  Discrete-Time Integrator6/1 -> MATLAB Function/2(wInt)
  "z "/1 -> MATLAB Function/1(Alt)
  Signal Builder6/1(Blender) -> MATLAB Function/3(x)
  [vW] -> "y "/1
  [vK] -> "y "/2
  "y "/1 -> Discrete-Time Integrator1/1
  Sum9/1 -> Gain29/1, "psi "/1
  Sum14/1 -> Gain30/1, "r "/1
  "u "/1 -> Sum15/2
  "theta "/1 -> Manual Switch14/1
  [uK] -> "u "/2
  "x "/1 -> Discrete-Time Integrator/1
  Sum15/1 -> u/1, "u "/1
  Discrete-Time Integrator/1 -> Sum8/2
  [q] -> Sum16/2
  [thetaK] -> "theta "/2
  [uW] -> "u "/1
  [thetaW] -> "theta "/1
  [uK] -> "x "/2
  [uW] -> "x "/1
  theta/1 -> To Workspace8/1, Sum1/1
  "q "/1 -> To Workspace9/1, Sum1/2
  x/1 -> To Workspace10/1, Sum1/3
  u/1 -> To Workspace11/1, Sum1/4
  Discrete Derivative/1 -> Switch1/2
  z/1 -> Switch1/3
  Sum8/1 -> x/1, "x "/1
  Sum16/1 -> "q "/1, "q "/1
  "theta "/1 -> Manual Switch14/2
  Sum17/1 -> theta/1, "theta "/1
  Manual Switch14/1 -> Sum17/2
  Sum18/1 -> w/1, "w "/1
  "phi "/1 -> Manual Switch3/2
  Manual Switch3/1 -> Sum19/2
  Sum19/1 -> phi/1, "phi "/1
  Sum20/1 -> "p "/1, "p "/1
  Sum21/1 -> v/1, "v "/1
  Sum22/1 -> y/1, "y "/1
  [wControl] -> Sum18/1
  [zControl] -> Sum10/1
  [thetaControl] -> Sum17/1
  [qControl] -> Sum16/1
  [xControl] -> Sum8/1
  [uControl] -> Sum15/1
  [phiControl] -> Sum19/1
  [pControl] -> Sum20/1
  [yControl] -> Sum22/1
  [vControl] -> Sum21/1
  [psiControl] -> Sum9/1
  [rControl] -> Sum14/1
  Sum2/1 -> Sum12/2
  Constant2/1 -> Switch1/1
  SystemID BangBang/1(Signal 1) -> Sum5/1
  SystemID BangBang/2(Signal 2) -> Sum5/2
  Constant1/1 -> Sum11/1
  Constant/1 -> Sum12/1
  [BangBang] -> Sum6/3

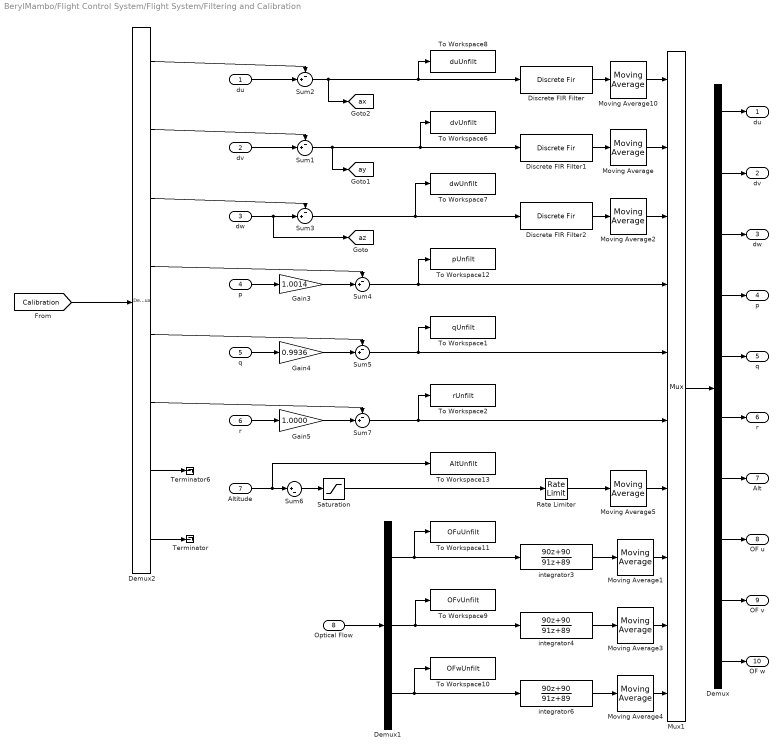
== system BerylMambo/Flight Control System/Flight System/Filtering and Calibration ==
  du : Inport
  dv : Inport  Port=2
  dw : Inport  Port=3
  p : Inport  Port=4
  q : Inport  Port=5
  r : Inport  Port=6
  Altitude : Inport  Port=7
  Optical Flow : Inport  Port=8
  Demux : Demux  Outputs=10
  Demux1 : Demux  Outputs=3
  Demux2 : Demux  Outputs=8
  Discrete FIR Filter : DiscreteFir  Coefficients=|
      | [0.0264    0.1405    0.3331    0.3331    0.1405    0.0264
      | ]
  Discrete FIR Filter1 : DiscreteFir  Coefficients=|
      | [0.0264    0.1405    0.3331    0.3331    0.1405    0.0264
      | ]
  Discrete FIR Filter2 : DiscreteFir  Coefficients=|
      | [0.0264    0.1405    0.3331    0.3331    0.1405    0.0264
      | ]
  Gain3 : Gain  Gain=1.0014
  Gain4 : Gain  Gain=0.9936
  Gain5 : Gain  Gain=1.0000
  Moving Average : dspstat3/Moving Average  Method=Exponential weighting  ForgettingFactorPort=off  SpecifyWindowLength=on  WindowLength=600  ForgettingFactor=0.2  SimulateUsing=Code generation
  Moving Average1 : dspstat3/Moving Average  Method=Exponential weighting  ForgettingFactorPort=off  SpecifyWindowLength=on  WindowLength=250  ForgettingFactor=0.5  SimulateUsing=Code generation
  Moving Average10 : dspstat3/Moving Average  Method=Exponential weighting  ForgettingFactorPort=off  SpecifyWindowLength=on  WindowLength=5  ForgettingFactor=0.2  SimulateUsing=Code generation
  Moving Average2 : dspstat3/Moving Average  Method=Exponential weighting  ForgettingFactorPort=off  SpecifyWindowLength=on  WindowLength=250  ForgettingFactor=0.2  SimulateUsing=Code generation
  Moving Average3 : dspstat3/Moving Average  Method=Exponential weighting  ForgettingFactorPort=off  SpecifyWindowLength=on  WindowLength=250  ForgettingFactor=0.5  SimulateUsing=Code generation
  Moving Average4 : dspstat3/Moving Average  Method=Exponential weighting  ForgettingFactorPort=off  SpecifyWindowLength=on  WindowLength=250  ForgettingFactor=0.5  SimulateUsing=Code generation
  Moving Average5 : dspstat3/Moving Average  Method=Sliding window  ForgettingFactorPort=off  SpecifyWindowLength=on  WindowLength=50  ForgettingFactor=0.5  SimulateUsing=Code generation
  Mux1 : Mux  Inputs=10
  Rate Limiter : RateLimiter  RisingSlewLimit=0.5  FallingSlewLimit=-0.5  SampleTimeMode=inherited
  Saturation : Saturate  UpperLimit=inf  LowerLimit=0  OutDataTypeStr=single
  Sum{1..5,7} (6 alike) : Sum  Inputs=-+|
  Sum6 : Sum  Inputs=|+-
  Terminator : Terminator
  Terminator6 : Terminator
  To Workspace1 : ToWorkspace  VariableName=qUnfilt  SaveFormat=Structure With Time  SampleTime=-1
  To Workspace10 : ToWorkspace  VariableName=OFwUnfilt  SaveFormat=Structure With Time  SampleTime=-1
  To Workspace11 : ToWorkspace  VariableName=OFuUnfilt  SaveFormat=Structure With Time  SampleTime=-1
  To Workspace12 : ToWorkspace  VariableName=pUnfilt  SaveFormat=Structure With Time  SampleTime=-1
  To Workspace13 : ToWorkspace  VariableName=AltUnfilt  SaveFormat=Structure With Time  SampleTime=-1
  To Workspace2 : ToWorkspace  VariableName=rUnfilt  SaveFormat=Structure With Time  SampleTime=-1
  To Workspace6 : ToWorkspace  VariableName=dvUnfilt  SaveFormat=Structure With Time  SampleTime=-1
  To Workspace7 : ToWorkspace  VariableName=dwUnfilt  SaveFormat=Structure With Time  SampleTime=-1
  To Workspace8 : ToWorkspace  VariableName=duUnfilt  SaveFormat=Structure With Time  SampleTime=-1
  To Workspace9 : ToWorkspace  VariableName=OFvUnfilt  SaveFormat=Structure With Time  SampleTime=-1
  integrator3 : DiscreteTransferFcn  Numerator=[90 90]  Denominator=[91 89]
  integrator4 : DiscreteTransferFcn  Numerator=[90 90]  Denominator=[91 89]
  integrator6 : DiscreteTransferFcn  Numerator=[90 90]  Denominator=[91 89]
  "du " : Outport
  "dv " : Outport  Port=2
  "dw " : Outport  Port=3
  "p " : Outport  Port=4
  "q " : Outport  Port=5
  "r " : Outport  Port=6
  Alt : Outport  Port=7
  "OF u " : Outport  Port=8
  "OF v " : Outport  Port=9
  "OF w " : Outport  Port=10
  tag scope: ax=global, ay=global, az=global
  wires:
  Demux/7 -> Alt/1
  Demux/2 -> "dv "/1
  Demux/3 -> "dw "/1
  Demux/1 -> "du "/1
  Mux1/1 -> Demux/1
  p/1 -> Gain3/1
  q/1 -> Gain4/1
  r/1 -> Gain5/1
  Sum1/1 -> Discrete FIR Filter1/1, To Workspace6/1, [ay]
  Sum2/1 -> Discrete FIR Filter/1, To Workspace8/1, [ax]
  Sum3/1 -> Discrete FIR Filter2/1, To Workspace7/1
  Demux/5 -> "q "/1
  Demux/4 -> "p "/1
  Demux/6 -> "r "/1
  Sum4/1 -> Mux1/4, To Workspace12/1
  Sum5/1 -> Mux1/5, To Workspace1/1
  Sum7/1 -> Mux1/6, To Workspace2/1
  du/1 -> Sum2/2
  dv/1 -> Sum1/2
  dw/1 -> [az], Sum3/2
  Gain3/1 -> Sum4/2
  Gain4/1 -> Sum5/2
  Gain5/1 -> Sum7/2
  Sum6/1 -> Saturation/1
  Optical Flow/1 -> Demux1/1
  Demux/8 -> "OF u "/1
  Demux/9 -> "OF v "/1
  Demux/10 -> "OF w "/1
  [Calibration] -> Demux2/1
  Demux2/1 -> Sum2/1
  Demux2/2 -> Sum1/1
  Demux2/3 -> Sum3/1
  Demux2/4 -> Sum4/1
  Demux2/5 -> Sum5/1
  Demux2/6 -> Sum7/1
  Demux2/7 -> Terminator6/1
  integrator3/1 -> Moving Average1/1
  integrator4/1 -> Moving Average3/1
  integrator6/1 -> Moving Average4/1
  Demux1/2 -> To Workspace9/1, integrator4/1
  Demux1/1 -> To Workspace11/1, integrator3/1
  Demux1/3 -> To Workspace10/1, integrator6/1
  Moving Average1/1 -> Mux1/8
  Moving Average3/1 -> Mux1/9
  Moving Average4/1 -> Mux1/10
  Discrete FIR Filter2/1 -> Moving Average2/1
  Discrete FIR Filter/1 -> Moving Average10/1
  Discrete FIR Filter1/1 -> Moving Average/1
  Moving Average2/1 -> Mux1/3
  Moving Average/1 -> Mux1/2
  Moving Average10/1 -> Mux1/1
  Saturation/1 -> Rate Limiter/1
  Moving Average5/1 -> Mux1/7
  Demux2/8 -> Terminator/1
  Rate Limiter/1 -> Moving Average5/1
  Altitude/1 -> To Workspace13/1, Sum6/1

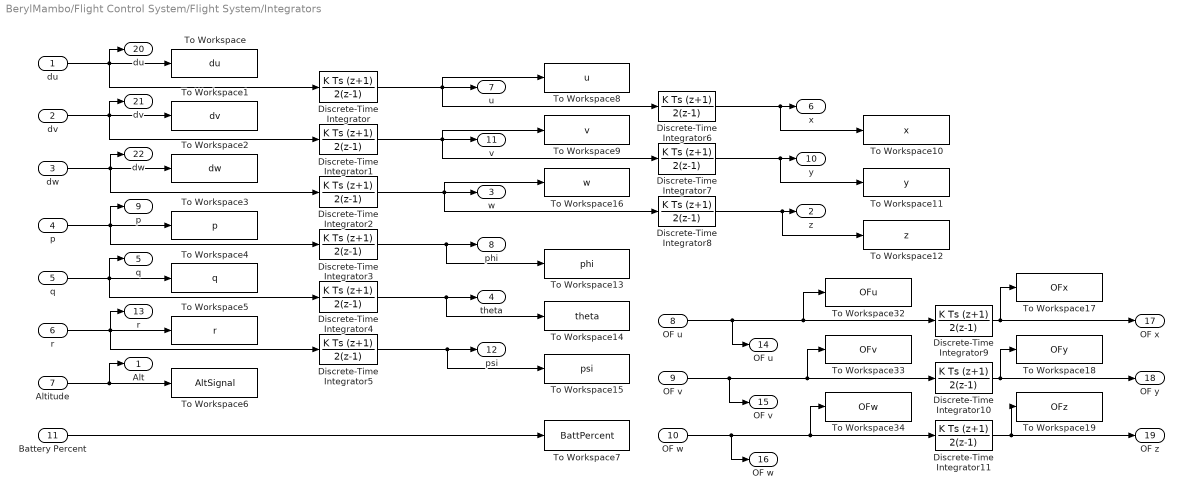
== system BerylMambo/Flight Control System/Flight System/Integrators ==
  du : Inport
  dv : Inport  Port=2
  dw : Inport  Port=3
  p : Inport  Port=4
  q : Inport  Port=5
  r : Inport  Port=6
  Altitude : Inport  Port=7
  "OF u " : Inport  Port=8
  "OF v " : Inport  Port=9
  "OF w " : Inport  Port=10
  Battery Percent : Inport  Port=11
  Discrete-Time Integrator{,1..5,8,11} (8 alike) : DiscreteIntegrator  IntegratorMethod=Integration: Trapezoidal  SampleTime=1/200  ICPrevOutput=DiscIntNeverNeededParam  ICPrevScaledInput=DiscIntNeverNeededParam
  Discrete-Time Integrator{6..7,9..10} (4 alike) : DiscreteIntegrator  IntegratorMethod=Integration: Trapezoidal  gainval=1  SampleTime=1/200  ICPrevOutput=DiscIntNeverNeededParam  ICPrevScaledInput=DiscIntNeverNeededParam
  To Workspace : ToWorkspace  VariableName=du  SaveFormat=Structure With Time  SampleTime=-1
      settings: MaxDataPoints=Inf
  To Workspace1 : ToWorkspace  VariableName=dv  SaveFormat=Structure With Time  SampleTime=-1
      settings: MaxDataPoints=Inf
  To Workspace10 : ToWorkspace  VariableName=x  SaveFormat=Structure With Time  SampleTime=-1
      settings: MaxDataPoints=Inf
  To Workspace11 : ToWorkspace  VariableName=y  SaveFormat=Structure With Time  SampleTime=-1
      settings: MaxDataPoints=Inf
  To Workspace12 : ToWorkspace  VariableName=z  SaveFormat=Structure With Time  SampleTime=-1
      settings: MaxDataPoints=Inf
  To Workspace13 : ToWorkspace  VariableName=phi  SaveFormat=Structure With Time  SampleTime=-1
      settings: MaxDataPoints=Inf
  To Workspace14 : ToWorkspace  VariableName=theta  SaveFormat=Structure With Time  SampleTime=-1
      settings: MaxDataPoints=Inf
  To Workspace15 : ToWorkspace  VariableName=psi  SaveFormat=Structure With Time  SampleTime=-1
      settings: MaxDataPoints=Inf
  To Workspace16 : ToWorkspace  VariableName=w  SaveFormat=Structure With Time  SampleTime=-1
      settings: MaxDataPoints=Inf
  To Workspace17 : ToWorkspace  VariableName=OFx  SaveFormat=Structure With Time  SampleTime=-1
      settings: MaxDataPoints=Inf
  To Workspace18 : ToWorkspace  VariableName=OFy  SaveFormat=Structure With Time  SampleTime=-1
      settings: MaxDataPoints=Inf
  To Workspace19 : ToWorkspace  VariableName=OFz  SaveFormat=Structure With Time  SampleTime=-1
      settings: MaxDataPoints=Inf
  To Workspace2 : ToWorkspace  VariableName=dw  SaveFormat=Structure With Time  SampleTime=-1
      settings: MaxDataPoints=Inf
  To Workspace3 : ToWorkspace  VariableName=p  SaveFormat=Structure With Time  SampleTime=-1
      settings: MaxDataPoints=Inf
  To Workspace32 : ToWorkspace  VariableName=OFu  SaveFormat=Structure With Time  SampleTime=-1
      settings: MaxDataPoints=Inf
  To Workspace33 : ToWorkspace  VariableName=OFv  SaveFormat=Structure With Time  SampleTime=-1
      settings: MaxDataPoints=Inf
  To Workspace34 : ToWorkspace  VariableName=OFw  SaveFormat=Structure With Time  SampleTime=-1
      settings: MaxDataPoints=Inf
  To Workspace4 : ToWorkspace  VariableName=q  SaveFormat=Structure With Time  SampleTime=-1
      settings: MaxDataPoints=Inf
  To Workspace5 : ToWorkspace  VariableName=r  SaveFormat=Structure With Time  SampleTime=-1
      settings: MaxDataPoints=Inf
  To Workspace6 : ToWorkspace  VariableName=AltSignal  SaveFormat=Structure With Time  SampleTime=-1
      settings: MaxDataPoints=Inf
  To Workspace7 : ToWorkspace  VariableName=BattPercent  SaveFormat=Structure With Time  SampleTime=-1
  To Workspace8 : ToWorkspace  VariableName=u  SaveFormat=Structure With Time  SampleTime=-1
      settings: MaxDataPoints=Inf
  To Workspace9 : ToWorkspace  VariableName=v  SaveFormat=Structure With Time  SampleTime=-1
      settings: MaxDataPoints=Inf
  "Alt " : Outport
  "z " : Outport  Port=2
  "w " : Outport  Port=3
  "theta " : Outport  Port=4
  "q " : Outport  Port=5
  "x " : Outport  Port=6
  "u " : Outport  Port=7
  "phi " : Outport  Port=8
  "p " : Outport  Port=9
  "y " : Outport  Port=10
  "v " : Outport  Port=11
  "psi " : Outport  Port=12
  "r " : Outport  Port=13
  OF u : Outport  Port=14
  "OF v " : Outport  Port=15
  OF w : Outport  Port=16
  "OF x " : Outport  Port=17
  "OF y " : Outport  Port=18
  "OF z " : Outport  Port=19
  "du " : Outport  Port=20
  "dv " : Outport  Port=21
  "dw " : Outport  Port=22
  wires:
  Discrete-Time Integrator4/1 -> To Workspace14/1, "theta "/1
  Discrete-Time Integrator5/1 -> To Workspace15/1, "psi "/1
  Altitude/1 -> To Workspace6/1, "Alt "/1
  Discrete-Time Integrator3/1 -> To Workspace13/1, "phi "/1
  Battery Percent/1 -> To Workspace7/1
  du/1 -> "du "/1, To Workspace/1, Discrete-Time Integrator/1
  p/1 -> Discrete-Time Integrator3/1, "p "/1, To Workspace3/1
  q/1 -> Discrete-Time Integrator4/1, "q "/1, To Workspace4/1
  r/1 -> Discrete-Time Integrator5/1, "r "/1, To Workspace5/1
  Discrete-Time Integrator/1 -> Discrete-Time Integrator6/1, To Workspace8/1, "u "/1
  Discrete-Time Integrator1/1 -> "v "/1, Discrete-Time Integrator7/1, To Workspace9/1
  Discrete-Time Integrator2/1 -> To Workspace16/1, Discrete-Time Integrator8/1, "w "/1
  dv/1 -> To Workspace1/1, Discrete-Time Integrator1/1, "dv "/1
  "OF w "/1 -> OF w/1, To Workspace34/1, Discrete-Time Integrator11/1
  dw/1 -> "dw "/1, Discrete-Time Integrator2/1, To Workspace2/1
  Discrete-Time Integrator6/1 -> "x "/1, To Workspace10/1
  Discrete-Time Integrator7/1 -> "y "/1, To Workspace11/1
  Discrete-Time Integrator8/1 -> To Workspace12/1, "z "/1
  Discrete-Time Integrator9/1 -> To Workspace17/1, "OF x "/1
  Discrete-Time Integrator10/1 -> To Workspace18/1, "OF y "/1
  Discrete-Time Integrator11/1 -> To Workspace19/1, "OF z "/1
  "OF u "/1 -> OF u/1, To Workspace32/1, Discrete-Time Integrator9/1
  "OF v "/1 -> "OF v "/1, To Workspace33/1, Discrete-Time Integrator10/1

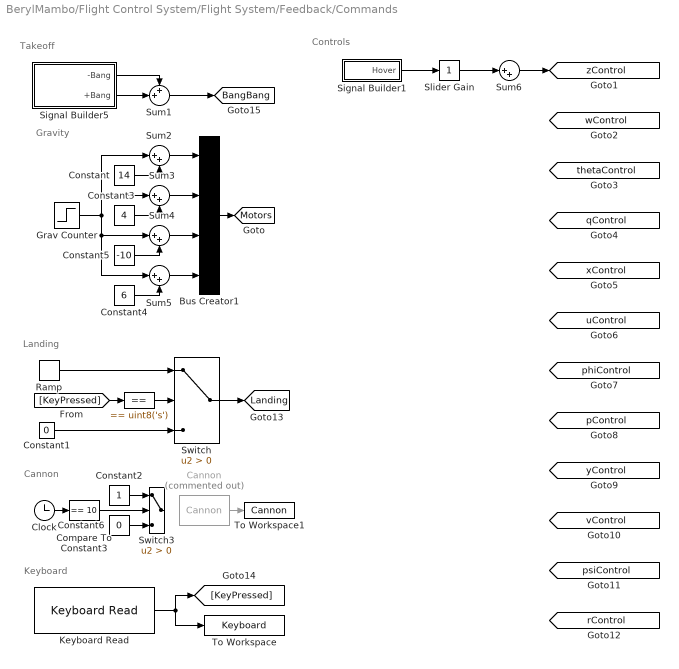
== system BerylMambo/Flight Control System/Flight System/Feedback/Commands  ==
  note: Keyboard
  note: Controls
  note: Cannon
  note: Takeoff
  note: Landing
  note: Gravity
  " " : simulink/Logic and Bit Operations/Compare To Constant  relop===  const=uint8('s')  OutDataTypeStr=boolean
  Bus Creator1 : BusCreator  Inputs=4
  Cannon : parrotlib/Cannon  Commented=on
      settings: SourceProductName=Simulink Support Package for Parrot Minidrones  SourceProductBaseCode=MINIDRONES
  Clock : Clock
  Compare To Constant3 : simulink/Logic and Bit Operations/Compare To Constant  relop===  const=10  OutDataTypeStr=boolean
  Constant : Constant  Value=14
  Constant1 : Constant  Value=0
  Constant2 : Constant
  Constant3 : Constant  Value=4
  Constant4 : Constant  Value=6
  Constant5 : Constant  Value=-10
  Constant6 : Constant  Value=0
  Grav Counter : Step  After=291  SampleTime=0
  Keyboard Read : parrotlib/Keyboard Read  SampleTime_=0.005
      settings: SourceProductName=Simulink Support Package for Parrot Minidrones  SourceProductBaseCode=MINIDRONES
  Ramp : simulink/Sources/Ramp  slope=-60  start=15  InitialOutput=0  VectorParams1D=off
  Signal Builder1 : Subsystem  Tag=STV Subsys  LoadFcn=sigbuilder_block('load');  StartFcn=sigbuilder_block('start');  StopFcn=sigbuilder_block('stop');  ClipboardFcn=sigbuilder_block('clipboard');  mask(Sigbuilder block){tuvar=[0:10]}
      mask help: Simulink:masks:SigbuilderBlock_MD
      mask init:
      | if ~strcmp(get_param(bdroot(gcbh),'SimulationStatus'),'stopped') tuvar = sigbuilder_block('maskInit'); end
      settings: CopyFcn=sigbuilder_block('copy');  DeleteFcn=sigbuilder_block('delete');  ModelCloseFcn=sigbuilder_block('modelClose');  PreSaveFcn=sigbuilder_block('preSave');  PauseFcn=sigbuilder_block('pause');  ContinueFcn=sigbuilder_block('continue');  NameChangeFcn=sigbuilder_block('namechange');  OpenFcn=sigbuilder_block('open',[0 51 1440 753 ]);  CloseFcn=sigbuilder_block('close');
      mask Display: plot(0, 0, 100, 100,[2, 2, 32, 32, 2], [68, 8, 8, 68, 68],[32, 2], [38, 38], [32, 19, 2],[53, 60, 44], [32, 17, 17, 2],[16, 16, 31, 31]);txt = getActiveGroup(gcbh);text(2, 100, txt,'verticalAlignment', 'top');
  Signal Builder5 : Subsystem  Tag=STV Subsys  LoadFcn=sigbuilder_block('load');  StartFcn=sigbuilder_block('start');  StopFcn=sigbuilder_block('stop');  ClipboardFcn=sigbuilder_block('clipboard');  mask(Sigbuilder block){tuvar=[0:10]}
      mask help: Simulink:masks:SigbuilderBlock_MD
      mask init:
      | if ~strcmp(get_param(bdroot(gcbh),'SimulationStatus'),'stopped') tuvar = sigbuilder_block('maskInit'); end
      settings: CopyFcn=sigbuilder_block('copy');  DeleteFcn=sigbuilder_block('delete');  ModelCloseFcn=sigbuilder_block('modelClose');  PreSaveFcn=sigbuilder_block('preSave');  PauseFcn=sigbuilder_block('pause');  ContinueFcn=sigbuilder_block('continue');  NameChangeFcn=sigbuilder_block('namechange');  OpenFcn=sigbuilder_block('open',[153 118 1287 686 ]);  CloseFcn=sigbuilder_block('close');
      mask Display: plot(0, 0, 100, 100,[2, 2, 32, 32, 2], [68, 8, 8, 68, 68],[32, 2], [38, 38], [32, 19, 2],[53, 60, 44], [32, 17, 17, 2],[16, 16, 31, 31]);txt = getActiveGroup(gcbh);text(2, 100, txt,'verticalAlignment', 'top');
  Slider Gain : simulink/Math Operations/Slider Gain  gain=1  low=-2  high=2
  Sum1 : Sum  Inputs=++|  OutDataTypeStr=single
  Sum{2..5} (4 alike) : Sum  Inputs=|++
  Sum6 : Sum  Inputs=|++  AccumDataTypeStr=single
  Switch : Switch  Criteria=u2 > Threshold  OutDataTypeStr=single
  Switch3 : Switch  Criteria=u2 > Threshold
  To Workspace : ToWorkspace  VariableName=Keyboard  SaveFormat=Structure  SampleTime=-1
  To Workspace1 : ToWorkspace  VariableName=Cannon  SaveFormat=Timeseries  SampleTime=-1
  tag scope: BangBang=global, Landing=global, Motors=global, pControl=global, phiControl=global, psiControl=global, qControl=global, rControl=global, thetaControl=global, uControl=global, vControl=global, wControl=global, xControl=global, yControl=global, zControl=global
  wires:
  Sum3/1 -> Bus Creator1/2
  Sum2/1 -> Bus Creator1/1
  Sum4/1 -> Bus Creator1/3
  Grav Counter/1 -> Sum5/1, Sum4/1, Sum3/1, Sum2/1
  Sum5/1 -> Bus Creator1/4
  " "/1 -> Switch/2
  Signal Builder5/2(+Bang) -> Sum1/2
  Signal Builder5/1(-Bang) -> Sum1/1
  Bus Creator1/1 -> [Motors]
  Constant1/1 -> Switch/3
  Signal Builder1/1(Hover) -> Slider Gain/1
  Slider Gain/1 -> Sum6/1
  [KeyPressed] -> " "/1
  Keyboard Read/1 -> To Workspace/1, [KeyPressed]
  Clock/1 -> Compare To Constant3/1
  Compare To Constant3/1 -> Switch3/2
  Cannon/1 -> To Workspace1/1
  Constant2/1 -> Switch3/1
  Constant6/1 -> Switch3/3
  Constant/1 -> Sum2/2
  Constant5/1 -> Sum4/2
  Sum1/1 -> [BangBang]
  Sum6/1 -> [zControl]
  Switch/1 -> [Landing]
  Ramp/1 -> Switch/1
  Constant4/1 -> Sum5/2
  Constant3/1 -> Sum3/2

== system BerylMambo/Flight Control System/Flight System/Feedback/Signal Builder6 ==
  Demux : Demux  Tag=STV Demux  Outputs=1
  FromWs : FromWorkspace  Tag=STV FromWs  VariableName=tuvar  SampleTime=0
      SigBuilderData=|
      | common.afterFinalStr = 'Extrapolate'
      | common.sampleTime = 0
      | dataSet.timeRange = [0 10]
      | dataSet.name = ' '
      | sbobj.Groups.Name = ' '
      | sbobj.Groups.Signals.Name = 'Blender'
      | sbobj.Groups.Signals.XData = [0 2 5 7 10]
      | sbobj.Groups.Signals.YData = [1 1 0.1 0 0]
  Blender : Outport  Tag=STV Outport
  wires:
  Demux/1 -> Blender/1
  FromWs/1 -> Demux/1

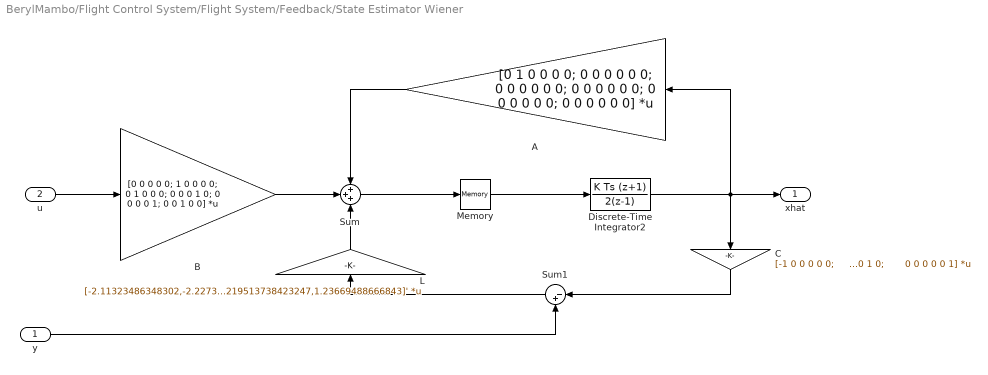
== system BerylMambo/Flight Control System/Flight System/Feedback/State Estimator Wiener  ==
  y : Inport
  u : Inport  Port=2
  A : Gain  Gain=|  Multiplication=Matrix(K*u)
      | [0 1 0 0 0 0;
      |      0 0 0 0 0 0;
      |      0 0 0 0 0 0;
      |      0 0 0 0 0 0;
      |      0 0 0 0 0 0;
      |      0 0 0 0 0 0]
  B : Gain  Gain=|  Multiplication=Matrix(K*u)
      | [0 0 0 0 0;
      |      1 0 0 0 0;
      |      0 1 0 0 0;
      |      0 0 0 1 0;
      |      0 0 0 0 1;
      |      0 0 1 0 0]
  C : Gain  Gain=|  Multiplication=Matrix(K*u)
      | [-1 0 0 0 0 0;
      |       0 0 1 0 0 0;
      |       0 0 0 1 0 0;
      |       0 0 0 0 1 0;
      |       0 0 0 0 0 1]
  Discrete-Time Integrator2 : DiscreteIntegrator  IntegratorMethod=Integration: Trapezoidal  SampleTime=1/200  ICPrevOutput=DiscIntNeverNeededParam  ICPrevScaledInput=DiscIntNeverNeededParam
  L : Gain  Gain=[-2.11323486348302,-2.22733357085530,-0.00616699432047580,-0.0589435329280187,-0.0380301004246628,0.00270456723382453;-0.0613701380466337,-0.464990419576037,3.76829194055976,-0.706565255779016,-0.0146674059755711,0.0560996319938339;3.46979348102631e-06,8.72563530618991e-06,-1.48249998633841e-05,0.0199715162029237,-0.000160063980343302,-3.50969847419283e-05;0.000239621969801616,0.000287268642123274,-0.000284768859542952,-0.000235406868600884,0.00612251378813491,-3.61807049590389e-05;-0.0131423668857116,-0.0486925227071381,0.0800519271769244,0.494987969597668,-0.0219513738423247,1.23669488666843]'  Multiplication=Matrix(K*u)
  Memory : Memory
  Sum : Sum  Inputs=+++
  Sum1 : Sum  Inputs=|-+
  xhat : Outport
  wires:
  u/1 -> B/1
  B/1 -> Sum/2
  C/1 -> Sum1/1
  y/1 -> Sum1/2
  Sum1/1 -> L/1
  L/1 -> Sum/3
  A/1 -> Sum/1
  Sum/1 -> Memory/1
  Discrete-Time Integrator2/1 -> A/1, xhat/1, C/1
  Memory/1 -> Discrete-Time Integrator2/1

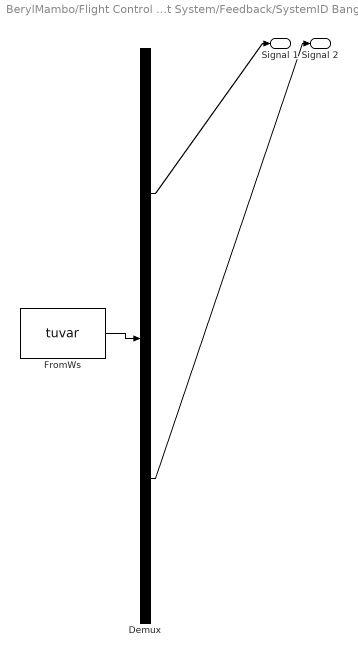
== system BerylMambo/Flight Control System/Flight System/Feedback/SystemID BangBang ==
  Demux : Demux  Tag=STV Demux  Outputs=2
  FromWs : FromWorkspace  Tag=STV FromWs  VariableName=tuvar  SampleTime=0
      SigBuilderData=|
      | common.afterFinalStr = 'Extrapolate'
      | common.sampleTime = 0
      | dataSet.timeRange = [0 10]
      | dataSet.name = 'Group 1'
      | sbobj.Groups.Name = 'Group 1'
      | sbobj.Groups.Signals(1).Name = 'Signal 1'
      | sbobj.Groups.Signals(1).XData = [0 6 6 6.5 6.5 10]
      | sbobj.Groups.Signals(1).YData = [0 0 40 40 0 0]
      | sbobj.Groups.Signals(2).Name = 'Signal 2'
      | sbobj.Groups.Signals(2).XData = [0 6.5 6.5 7 7 10]
      | sbobj.Groups.Signals(2).YData = [0 0 -40 -40 0 0]
  Signal 1 : Outport  Tag=STV Outport
  Signal 2 : Outport  Tag=STV Outport  Port=2
  wires:
  Demux/1 -> Signal 1/1
  Demux/2 -> Signal 2/1
  FromWs/1 -> Demux/1

== system BerylMambo/Flight Control System/Flight System/Feedback/Commands /Signal Builder1 ==
  Demux : Demux  Tag=STV Demux  Outputs=1
  FromWs : FromWorkspace  Tag=STV FromWs  VariableName=tuvar  SampleTime=0
      SigBuilderData=|
      | common.afterFinalStr = 'Extrapolate'
      | common.sampleTime = 0
      | dataSet.timeRange = [0 60]
      | dataSet.name = ' '
      | sbobj.Groups.Name = ' '
      | sbobj.Groups.Signals.Name = 'Hover'
      | sbobj.Groups.Signals.XData = [0 0.05 1.5 60]
      | sbobj.Groups.Signals.YData = [0 0 1 1]
      | sbobj.Groups.TimeRange = [0 60]
  Hover : Outport  Tag=STV Outport
  wires:
  FromWs/1 -> Demux/1
  Demux/1 -> Hover/1

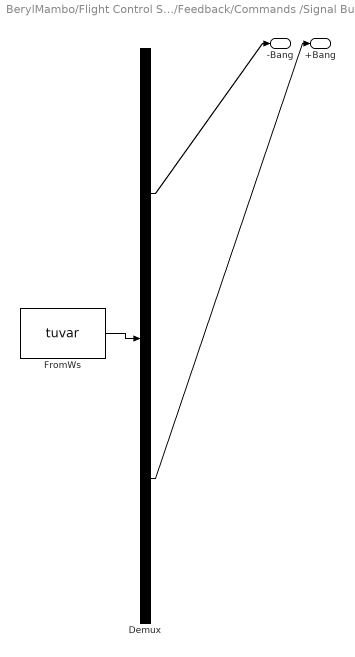
== system BerylMambo/Flight Control System/Flight System/Feedback/Commands /Signal Builder5 ==
  Demux : Demux  Tag=STV Demux  Outputs=2
  FromWs : FromWorkspace  Tag=STV FromWs  VariableName=tuvar  SampleTime=0
      SigBuilderData=|
      | common.afterFinalStr = 'Extrapolate'
      | common.sampleTime = 0
      | dataSet.timeRange = [0 10]
      | dataSet.name = 'Bang Bang'
      | sbobj.Groups.Name = 'Bang Bang'
      | sbobj.Groups.Signals(1).Name = '-Bang'
      | sbobj.Groups.Signals(1).XData = [0 0.5 0.5 1.15 1.15 10]
      | sbobj.Groups.Signals(1).YData = [0 0 -70 -70 0 0]
      | sbobj.Groups.Signals(2).Name = '+Bang'
      | sbobj.Groups.Signals(2).XData = [0 1.15 1.15 1.5 1.5 10]
      | sbobj.Groups.Signals(2).YData = [0 0 40 40 0 0]
  -Bang : Outport  Tag=STV Outport
  +Bang : Outport  Tag=STV Outport  Port=2
  wires:
  Demux/1 -> -Bang/1
  Demux/2 -> +Bang/1
  FromWs/1 -> Demux/1

== matlab function BerylMambo/Flight Control System/Flight System/Feedback/MATLAB Function ==
  data: Alt input; z output; wInt input; x input
function z = fcn(Alt, wInt, x)
z = Alt*(1-x) + wInt*x;
